simulink model "Glideslope_controller"  (R2023a)
settings: Solver=VariableStepAuto  StartTime=0.0  StopTime=10.0  RelTol=1e-3
libraries: cstblocks x5
settings Model: Creator=anape  LastModifiedBy=anape

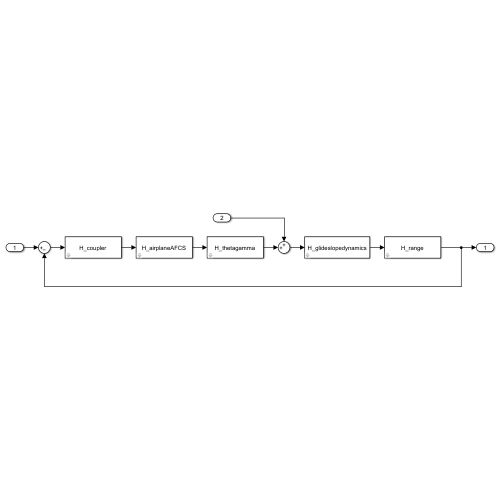
[thumbnail: Simulink's stored preview of the top-level diagram]
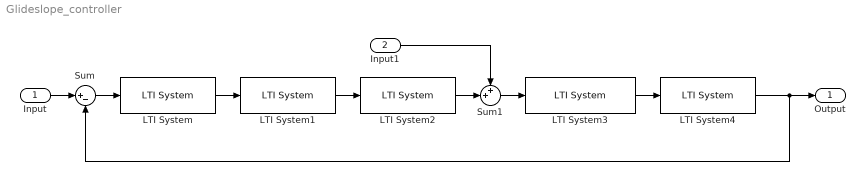
== system Glideslope_controller ==
  Input : Inport
  Input1 : Inport  Port=2
  LTI System : cstblocks/LTI System  sys=H_coupler  IC=[]
  LTI System1 : cstblocks/LTI System  sys=H_airplaneAFCS  IC=[]
  LTI System2 : cstblocks/LTI System  sys=tf(1,[1 1])  IC=[]
  LTI System3 : cstblocks/LTI System  sys=H_glideslopedynamics  IC=[]
  LTI System4 : cstblocks/LTI System  sys=H_range  IC=[]
  Sum : Sum  Inputs=|+-
  Sum1 : Sum  Inputs=++|
  Output : Outport
  wires:
  Input/1 -> Sum/1
  Sum/1 -> LTI System/1
  LTI System/1 -> LTI System1/1
  LTI System1/1 -> LTI System2/1
  LTI System2/1 -> Sum1/2
  Sum1/1 -> LTI System3/1
  LTI System3/1 -> LTI System4/1
  LTI System4/1 -> Sum/2, Output/1
  Input1/1 -> Sum1/1
